simulink model "LPV_MPC_1"  (R2020b)
settings: Solver=VariableStepAuto  StartTime=0.0  StopTime=11  MaxStep=Ts/2  RelTol=1e-3
values from neighbouring files (symbols this model uses):
  Cf = 117950    [LoadVehicleParameters.m]    (also in Pokreni.m = vehicle.Cf)
  Cr = 143700    [LoadVehicleParameters.m]    (also in Pokreni.m = vehicle.Cr)
  Csf = 0    [Pokreni.m]
  d = 0.793    [LoadVehicleParameters.m]    (also in Pokreni.m = vehicle.d)
  dlc = 0    [Pokreni.m]
  Iz = vehicle.Jz    [Pokreni.m]
  lf = 1.311    [LoadVehicleParameters.m]    (also in Pokreni.m = vehicle.lf)
  lr = 1.311    [LoadVehicleParameters.m]    (also in Pokreni.m = vehicle.lr)
  m = 1599.98    [LoadVehicleParameters.m]    (also in Pokreni.m = vehicle.m)
  md = getCurvature(v0,0:0.1:15)    [Pokreni.m]
  tau = 0.02    [Pokreni.m]
  Ts = 0.1    [Pokreni.m]
undefined symbols (not defined in the file or in its folder): nominalMPC
settings Model: Creator=Sandor  LastModifiedBy=LAMES Workstation
settings DebuggingCC: SFMachineParentedDataDiag=error

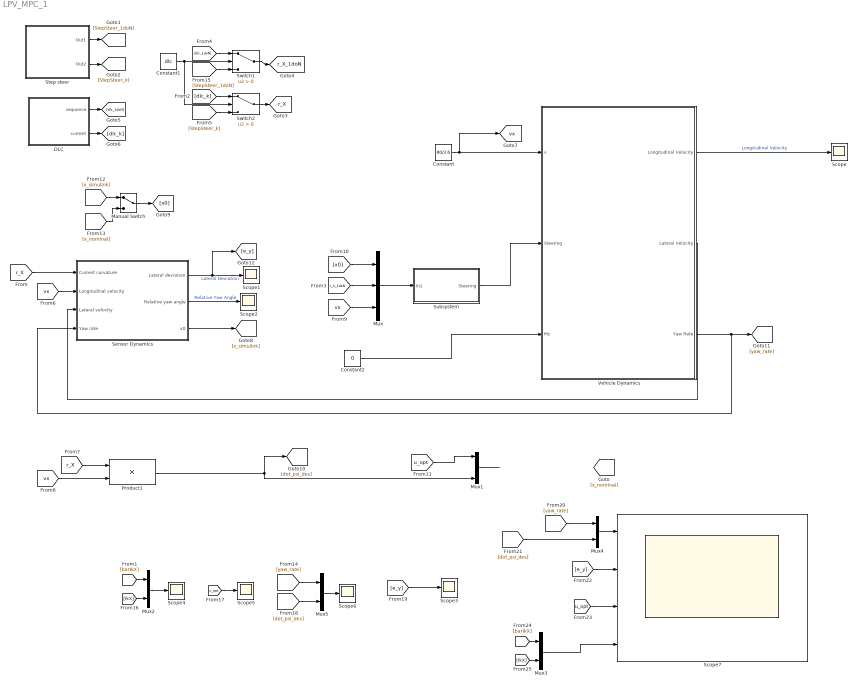
== system LPV_MPC_1 ==
  Constant : Constant  Value=80/3.6
  Constant1 : Constant  Value=dlc
  Constant2 : Constant  Value=0
  DLC : Subsystem  mask{signal=md, ts=Ts, steps=10}
      mask prompts: signal "Signal name"; ts "Sampling time"; steps "Number of previewing steps"
      mask init:
      | ts = evalin('base',get_param(gcbh,'ts'));
      | signal = evalin('base',get_param(gcbh,'signal'));
      | steps = evalin('base',get_param(gcbh,'steps'));
      | data = mpc_previewer_maskinit(signal,ts);
      mask Display:
      | fprintf('Future\nsample\nextractor');
      | port_label('output', 1, 'seq')
      | port_label('output', 2, '@t')
  Manual Switch : ManualSwitch
  Mux : Mux  Inputs=3
  Mux1 : Mux  Inputs=3
  Mux{2..5} (4 alike) : Mux  Inputs=2
  Product1 : Product
  Scope{,1..6} (7 alike) : Scope
  Scope7 : Scope  NumInputPorts=4
  Sensor Dynamics : Subsystem
  Step steer : Subsystem
  Subsystem : Subsystem
  Switch1 : Switch  Criteria=u2 > Threshold
  Switch2 : Switch  Criteria=u2 > Threshold
  Vehicle Dynamics : Subsystem
  tag scope: r_X=global, r_X_1doN=global, vx=global
  wires:
  Constant/1 -> [vx], Vehicle Dynamics/1(v)
  Vehicle Dynamics/1(Longitudinal Velocity) -> Scope/1  "Longitudinal Velocity"
  Vehicle Dynamics/2(Lateral Velocity) -> Sensor Dynamics/3(Lateral velocity)
  Vehicle Dynamics/3(Yaw Rate) -> [yaw_rate], Sensor Dynamics/4(Yaw rate)
  Sensor Dynamics/1(Lateral deviation) -> [e_y], Scope1/1  "Lateral Deviation"
  Sensor Dynamics/2(Relative yaw angle) -> Scope2/1  "Relative Yaw Angle"
  Mux1/1 -> ?
  [x0] -> Mux/1
  ? -> [x_nominal]
  [r_X] -> Sensor Dynamics/1(Current curvature)
  Product1/1 -> Mux1/3, [dot_psi_des]
  Step steer/1(Out1) -> [StepSteer_1doN]
  Step steer/2(Out2) -> [StepSteer_k]
  ? -> ?
  Switch2/1 -> [r_X]
  Switch1/1 -> [r_X_1doN]
  [r_X_1doN] -> Mux/2
  Constant1/1 -> Switch2/2, Switch1/2
  DLC/1(sequence) -> [dlc_1doN]
  DLC/2(current) -> [dlc_k]
  [vx] -> Sensor Dynamics/2(Longitudinal velocity)
  [r_X] -> Product1/1
  [vx] -> Product1/2
  [vx] -> Mux/3
  Sensor Dynamics/3(x0) -> [x_simulink]
  [x_simulink] -> Manual Switch/1
  [x_nominal] -> Manual Switch/2
  Manual Switch/1 -> [x0]
  [dlc_1doN] -> Switch1/1
  [StepSteer_1doN] -> Switch1/3
  [dlc_k] -> Switch2/1
  [StepSteer_k] -> Switch2/3
  [barIkX] -> Mux2/1
  [IkX] -> Mux2/2
  Mux2/1 -> Scope4/1
  [u_opt] -> Scope5/1
  [e_y] -> Scope3/1
  [yaw_rate] -> Mux4/1
  [dot_psi_des] -> Mux4/2
  Mux4/1 -> Scope7/1
  [e_y] -> Scope7/2
  [u_opt] -> Scope7/3
  [IkX] -> Mux3/2
  [barIkX] -> Mux3/1
  Mux3/1 -> Scope7/4
  [dot_psi_des] -> Mux5/2
  Mux5/1 -> Scope6/1
  [yaw_rate] -> Mux5/1
  Mux/1 -> Subsystem/1(In1)
  Subsystem/1(Steering) -> Vehicle Dynamics/2(Steering)
  Constant2/1 -> Vehicle Dynamics/3(Mz)
  [u_opt] -> Mux1/1

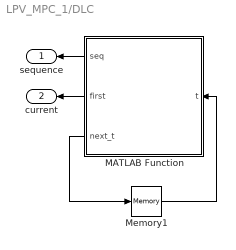
== system LPV_MPC_1/DLC ==
  MATLAB Function : MATLAB Function  TreatAsAtomicUnit=on
  Memory1 : Memory  InheritSampleTime=on  LinearizeAsDelay=on
  sequence : Outport  VectorParamsAs1DForOutWhenUnconnected=off
  current : Outport  Port=2  VectorParamsAs1DForOutWhenUnconnected=off
  wires:
  MATLAB Function/1(seq) -> sequence/1
  MATLAB Function/2(first) -> current/1
  Memory1/1 -> MATLAB Function/1(t)
  MATLAB Function/3(next_t) -> Memory1/1

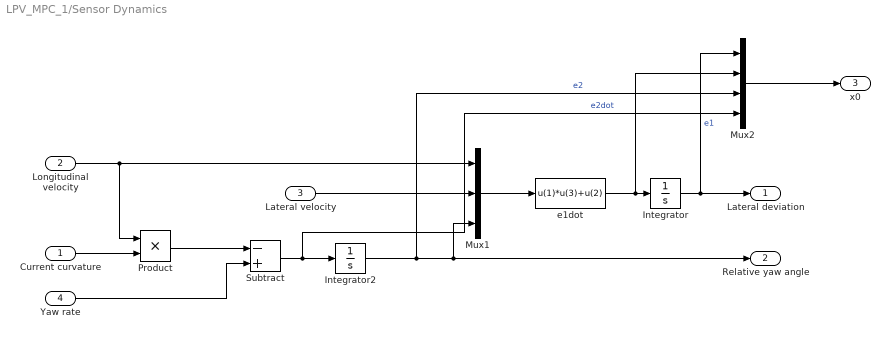
== system LPV_MPC_1/Sensor Dynamics ==
  Current curvature : Inport
  Longitudinal velocity : Inport  Port=2
  Lateral velocity : Inport  Port=3
  Yaw rate : Inport  Port=4
  Integrator : Integrator  InitialCondition=1
  Integrator2 : Integrator
  Mux1 : Mux  Inputs=[1 1 1]
  Mux2 : Mux
  Product : Product
  Subtract : Sum  Inputs=-+
  e1dot : Fcn  Expr=u(1)*u(3)+u(2)
  Lateral deviation : Outport  VectorParamsAs1DForOutWhenUnconnected=off
  Relative yaw angle : Outport  Port=2  VectorParamsAs1DForOutWhenUnconnected=off
  x0 : Outport  Port=3  VectorParamsAs1DForOutWhenUnconnected=off
  wires:
  Current curvature/1 -> Product/2
  Mux1/1 -> e1dot/1
  e1dot/1 -> Mux2/2, Integrator/1
  Longitudinal velocity/1 -> Product/1, Mux1/1
  Lateral velocity/1 -> Mux1/2
  Integrator/1 -> Mux2/1, Lateral deviation/1  "e1"
  Product/1 -> Subtract/1
  Yaw rate/1 -> Subtract/2
  Subtract/1 -> Mux2/4, Integrator2/1  "e2dot"
  Integrator2/1 -> Mux2/3, Mux1/3, Relative yaw angle/1  "e2"
  Mux2/1 -> x0/1

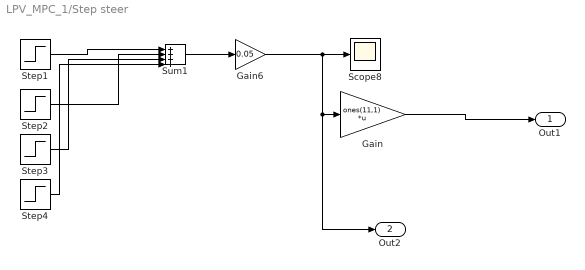
== system LPV_MPC_1/Step steer ==
  Gain : Gain  Gain=ones(11,1)  Multiplication=Matrix(K*u)
  Gain6 : Gain  Gain=0.05
  Scope8 : Scope
  Step1 : Step  SampleTime=0
  Step2 : Step  Time=3  After=-1  SampleTime=0
  Step3 : Step  Time=6  After=-1  SampleTime=0
  Step4 : Step  Time=9  SampleTime=0
  Sum1 : Sum  Inputs=|++++
  Out1 : Outport
  Out2 : Outport  Port=2
  wires:
  Gain6/1 -> Out2/1, Gain/1, Scope8/1
  Step4/1 -> Sum1/4
  Sum1/1 -> Gain6/1
  Step3/1 -> Sum1/3
  Step1/1 -> Sum1/1
  Step2/1 -> Sum1/2
  Gain/1 -> Out1/1

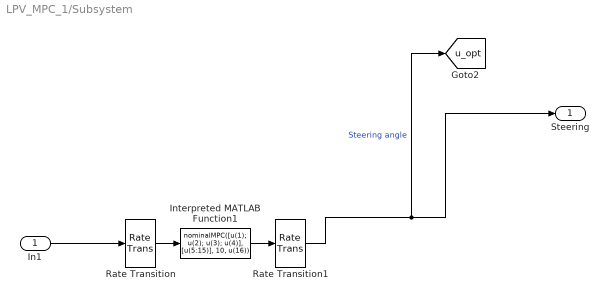
== system LPV_MPC_1/Subsystem ==
  In1 : Inport
  Interpreted MATLAB Function1 : MATLABFcn  MATLABFcn=nominalMPC([u(1); u(2); u(3); u(4)], [u(5:15)], 10, u(16))  OutputDimensions=1
  Rate Transition : RateTransition  OutPortSampleTime=0.1
  Rate Transition1 : RateTransition  OutPortSampleTime=0.1
  Steering : Outport
  tag scope: u_opt=global
  wires:
  Interpreted MATLAB Function1/1 -> Rate Transition1/1
  In1/1 -> Rate Transition/1
  Rate Transition/1 -> Interpreted MATLAB Function1/1
  Rate Transition1/1 -> [u_opt], Steering/1  "Steering angle"

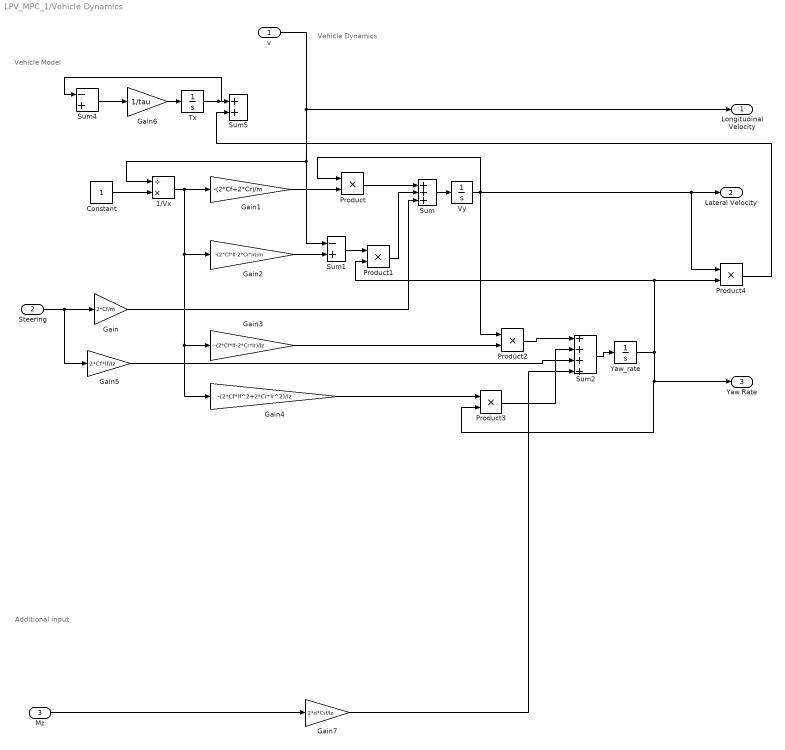
== system LPV_MPC_1/Vehicle Dynamics ==
  note: Vehicle Model
  note: Vehicle Dynamics
  note: Additional input
  v : Inport
  Steering : Inport  Port=2
  Mz : Inport  Port=3
  1/Vx : Product  Inputs=/*
  Constant : Constant
  Gain : Gain  Gain=2*Cf/m
  Gain1 : Gain  Gain=-(2*Cf+2*Cr)/m
  Gain2 : Gain  Gain=-(2*Cf*lf-2*Cr*lr)/m
  Gain3 : Gain  Gain=-(2*Cf*lf-2*Cr*lr)/Iz
  Gain4 : Gain  Gain=-(2*Cf*lf^2+2*Cr*lr^2)/Iz
  Gain5 : Gain  Gain=2*Cf*lf/Iz
  Gain6 : Gain  Gain=1/tau
  Gain7 : Gain  Gain=2*d*Csf/Iz
  Product{,1..4} (5 alike) : Product
  Sum : Sum  Inputs=+++
  Sum1 : Sum  Inputs=-+
  Sum2 : Sum  Inputs=++++
  Sum4 : Sum  Inputs=-+
  Sum5 : Sum
  Tx : Integrator
  Vy : Integrator
  "Yaw_rate " : Integrator
  Longitudinal Velocity : Outport  VectorParamsAs1DForOutWhenUnconnected=off
  Lateral Velocity : Outport  Port=2  VectorParamsAs1DForOutWhenUnconnected=off
  Yaw Rate : Outport  Port=3  VectorParamsAs1DForOutWhenUnconnected=off
  wires:
  Gain6/1 -> Tx/1
  Sum2/1 -> "Yaw_rate "/1
  Gain2/1 -> Sum1/2
  Gain4/1 -> Product3/1
  Constant/1 -> 1/Vx/2
  Gain3/1 -> Product2/2
  1/Vx/1 -> Gain4/1, Gain3/1, Gain2/1, Gain1/1
  Product2/1 -> Sum2/1
  Sum4/1 -> Gain6/1
  Tx/1 -> Sum4/1, Sum5/1
  Product3/1 -> Sum2/2
  Gain5/1 -> Sum2/3
  Product4/1 -> Sum5/2
  Sum1/1 -> Product1/1
  "Yaw_rate "/1 -> Yaw Rate/1, Product3/2, Product4/2, Product1/2
  Gain/1 -> Sum/3
  Steering/1 -> Gain/1, Gain5/1
  Gain1/1 -> Product/2
  Product/1 -> Sum/1
  Vy/1 -> Product/1, Lateral Velocity/1, Product4/1, Product2/1
  Sum/1 -> Vy/1
  v/1 -> Longitudinal Velocity/1, 1/Vx/1, Sum1/1
  Product1/1 -> Sum/2
  Mz/1 -> Gain7/1
  Gain7/1 -> Sum2/4

== matlab function LPV_MPC_1/DLC/MATLAB Function ==
  settings: updateMethod=DISCRETE  sampleTime=ts
  data: data parameter; seq output; steps parameter; t input; first output; next_t output
function [seq,first,next_t] = fcn(data,steps,t)
%#codegen
[seq,first,next_t] = mpcblock_preview('md',data,steps,t);
